simulink model "PWMepitettHidakhoz"  (R2013b)
settings: Solver=FixedStepDiscrete  SolverMode=SingleTasking  StartTime=0.0  StopTime=260000  FixedStep=0.1  RelTol=1e-3
undefined symbols (not defined in the file or in its folder): JA1, nexys2iroobo_lib
libraries: xbsIndex_r4 x41, simulink x2
settings Model: Creator=laca  LastModifiedBy=laca

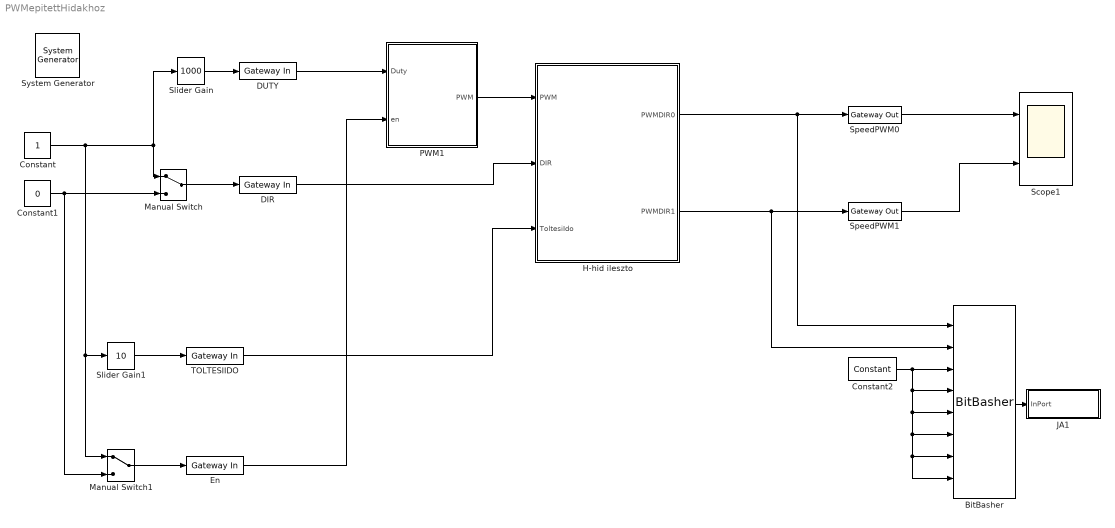
== system PWMepitettHidakhoz ==
  " System Generator" : xbsIndex_r4/ System Generator  Tag=genX  xilinxfamily=spartan3e  part=xc3s1200e  speed=-4  package=fg320  synthesis_tool=XST  clock_wrapper=Clock Enables  directory=./netlist  proj_type=Project Navigator  Synth_file=XST Defaults  Impl_file=ISE Defaults  testbench=off  simulink_period=1  sysclk_period=20  dcm_input_clock_period=10  incr_netlist=off  trim_vbits=Everywhere in SubSystem  dbl_ovrd=According to Block Masks  core_generation=According to Block Masks  run_coregen=off  deprecated_control=off  eval_field=0  block_type=sysgen
  BitBasher : xbsIndex_r4/BitBasher  bitexpr=|  display_expr=off  sr_1=1  arith_type1=Unsigned  bin_pt1=0  sr_2=2  arith_type2=Unsigned  bin_pt2=0  sr_3=3  arith_type3=Unsigned  bin_pt3=0  sr_4=4  arith_type4=Unsigned  bin_pt4=0  dbl_ovrd=off  block_type=bitbasher
      | <!DOCTYPE HTML PUBLIC "-//W3C//DTD HTML 4.0//EN" "http://www.w3.org/TR/REC-html40/strict.dtd">
      | <html><head><meta name="qrichtext" content="1" /><style type="text/css">
      | p, li { white-space: pre-wrap; }
      | </style></head><body style=" font-family:'MS Shell Dlg 2'; font-size:8.25pt; font-weight:400; font-style:normal;">
      | <p style=" margin-top:12px; margin-bottom:12px; margin-left:0px; margin-right:0px; -qt-block-indent:0; text-indent:0px;"><span style=" font-family:'MS Shell Dlg'; font-size:8pt;">a={b7,b6,b5,b4,b3,b2,b1,b0}</span></p></body></html>
  Constant : Constant
  Constant1 : Constant  Value=0
  Constant2 : xbsIndex_r4/Constant  const=0  gui_display_data_type=Boolean  arith_type=Boolean  n_bits=16  bin_pt=14  preci_type=Single  exp_width=8  frac_width=24  explicit_period=off  period=1  equ=P=C  opselect=C  inp2=PCIN>>17  opr=+  inp1=P  carry=CIN  dbl_ovrd=off  block_type=constant
  DIR : xbsIndex_r4/Gateway In  gui_display_data_type=Boolean  arith_type=Boolean  n_bits=16  bin_pt=0  preci_type=Single  exp_width=8  frac_width=24  quantization="Round  (unbiased: +/- Inf)"  overflow=Saturate  period=1  dbl_ovrd=off  timing_constraint=None  locs_specified=off  LOCs={}  UseAsADC=off  ADCChannel='1'  inherit_from_input=off  hdl_port=on  block_type=gatewayin
  DUTY : xbsIndex_r4/Gateway In  gui_display_data_type=Fixed-point  arith_type=Unsigned  n_bits=16  bin_pt=0  preci_type=Single  exp_width=8  frac_width=24  quantization="Round  (unbiased: +/- Inf)"  overflow=Saturate  period=1  dbl_ovrd=off  timing_constraint=None  locs_specified=off  LOCs={}  UseAsADC=off  ADCChannel='1'  inherit_from_input=off  hdl_port=on  block_type=gatewayin
  En : xbsIndex_r4/Gateway In  gui_display_data_type=Boolean  arith_type=Boolean  n_bits=16  bin_pt=14  preci_type=Single  exp_width=8  frac_width=24  quantization="Round  (unbiased: +/- Inf)"  overflow=Saturate  period=1  dbl_ovrd=off  timing_constraint=None  locs_specified=off  LOCs={}  UseAsADC=off  ADCChannel='1'  inherit_from_input=off  hdl_port=on  block_type=gatewayin
  H-hid ileszto : Subsystem
  JA1 : Subsystem  AncestorBlock=nexys2iroobo_lib/JA1  mask(Non-Memory-Mapped Output Port){show_out=off}
      mask prompts: show_out "Provide Output Double"
      mask help:
      | Port Name: "JA1"
      | Port Type: 8-bit Vector
      mask init:
      | [bg,fg] = xlcmap('IO',0);
      | iPos = get_param(gcb,'Position');
      | iWidth=iPos(3)-iPos(1);
      | iHeight=iPos(4)-iPos(2);
      | [logoX, logoY] = xlogo(iPos);
      | if (show_out)
      |     old = find_system(gcb, 'LookUnderMasks', 'all', 'Name', 'Terminator');
      |     if (length(old) > 0)
      |         replace_block(gcb, 'Name', 'Terminator', 'OutPort', 'noprompt');
      |         set_param([gcb '/Terminator'], 'Name', 'OutPort');
      |     end
      |     portdir = 'output';
      |     portstr = 'dbl';
      | else
      |     old = find_system(gcb, 'LookUnderMasks', 'all', 'name', 'OutPort');
      |     if (length(old) > 0)
      |         replace_block(gcb, 'Name', 'OutPort', 'Terminator', 'noprompt');
      |         set_param([gcb '/OutPort'], 'Name', 'Terminator');
      |     end
      |     portdir = 'input';
      |     portstr = '';
      | end
      settings: CopyFcn=set_param(gcb,'LinkStatus','inactive');
      mask Display:
      | patch([0 iWidth iWidth 0],[0 0 iHeight iHeight] , bg);
      | patch(logoX,logoY, fg);
      | plot([0 0 iWidth iWidth 0], [0 iHeight iHeight 0 0]);
      | port_label(portdir,1,portstr);
      | port_label('input',1,'JA1');
      | text(iWidth-10,5,'nmm');
  Manual Switch : ManualSwitch
  Manual Switch1 : ManualSwitch
  PWM1 : Subsystem
  Scope1 : Scope  NumInputPorts=2
      settings: TickLabels=on  ShowLegends=on  YMin=0~0  YMax=2000~1
  Slider Gain : simulink/Math Operations/Slider Gain  low=0  gain=1000  high=16535
  Slider Gain1 : simulink/Math Operations/Slider Gain  low=0  gain=10  high=1000
  SpeedPWM0 : xbsIndex_r4/Gateway Out  inherit_from_input=off  hdl_port=on  timing_constraint=None  locs_specified=off  LOCs={}  UseAsDAC=off  DACChannel='1'  block_type=gatewayout
      settings: xl_area=[0 0 0 0 1 0 0]
  SpeedPWM1 : xbsIndex_r4/Gateway Out  inherit_from_input=off  hdl_port=on  timing_constraint=None  locs_specified=off  LOCs={}  UseAsDAC=off  DACChannel='1'  block_type=gatewayout
      settings: xl_area=[0 0 0 0 1 0 0]
  TOLTESIIDO : xbsIndex_r4/Gateway In  gui_display_data_type=Fixed-point  arith_type=Unsigned  n_bits=16  bin_pt=0  preci_type=Single  exp_width=8  frac_width=24  quantization="Round  (unbiased: +/- Inf)"  overflow=Saturate  period=1  dbl_ovrd=off  timing_constraint=None  locs_specified=off  LOCs={}  UseAsADC=off  ADCChannel='1'  inherit_from_input=off  hdl_port=on  block_type=gatewayin
  wires:
  Manual Switch/1 -> DIR/1
  Slider Gain1/1 -> TOLTESIIDO/1
  TOLTESIIDO/1 -> H-hid ileszto/3(ToltesiIdo)
  Manual Switch1/1 -> En/1
  PWM1/1(PWM) -> H-hid ileszto/1(PWM)
  DIR/1 -> H-hid ileszto/2(DIR)
  H-hid ileszto/1(PWMDIR0) -> BitBasher/1, SpeedPWM0/1
  H-hid ileszto/2(PWMDIR1) -> BitBasher/2, SpeedPWM1/1
  En/1 -> PWM1/2(en)
  DUTY/1 -> PWM1/1(Duty)
  SpeedPWM0/1 -> Scope1/1
  SpeedPWM1/1 -> Scope1/2
  Slider Gain/1 -> DUTY/1
  Constant1/1 -> Manual Switch1/2, Manual Switch/2
  Constant/1 -> Slider Gain1/1, Manual Switch1/1, Slider Gain/1, Manual Switch/1
  BitBasher/1 -> JA1/1(InPort)
  Constant2/1 -> BitBasher/4, BitBasher/5, BitBasher/6, BitBasher/7, BitBasher/8, BitBasher/3

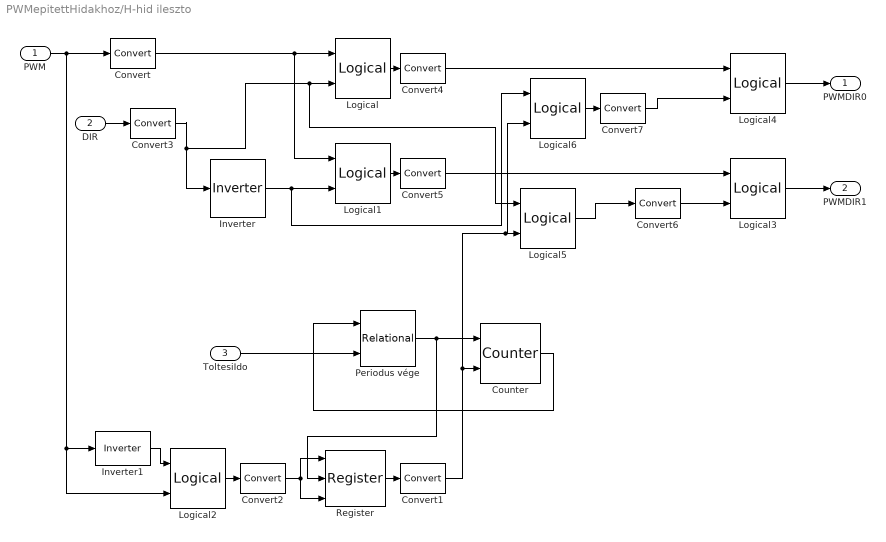
== system PWMepitettHidakhoz/H-hid ileszto ==
  PWM : Inport
  DIR : Inport  Port=2
  ToltesiIdo : Inport  Port=3
  Convert{,1..7} (8 alike) : xbsIndex_r4/Convert  gui_display_data_type=Boolean  arith_type=Boolean  n_bits=16  bin_pt=14  float_type=Single  exp_bits=8  fraction_bits=24  quantization=Truncate  overflow=Wrap  en=off  latency=0  dbl_ovrd=off  pipeline=off  block_type=convert
  Counter : xbsIndex_r4/Counter  cnt_type=Free Running  cnt_to=Inf  operation=Up  start_count=0  cnt_by_val=1  arith_type=Unsigned  n_bits=16  bin_pt=0  load_pin=off  rst=on  en=on  explicit_period=off  period=2*10^-2  dbl_ovrd=off  use_behavioral_HDL=off  implementation=Fabric  block_type=counter
  Inverter : xbsIndex_r4/Inverter  en=off  latency=0  dbl_ovrd=off  block_type=inv
  Inverter1 : xbsIndex_r4/Inverter  en=off  latency=1  dbl_ovrd=off  block_type=inv
  Logical{,1..2,5..6} (5 alike) : xbsIndex_r4/Logical  logical_function=AND  inputs=2  en=off  latency=0  precision=User Defined  arith_type=Unsigned  n_bits=1  bin_pt=0  align_bp=on  dbl_ovrd=off  block_type=logical
  Logical3 : xbsIndex_r4/Logical  logical_function=OR  inputs=2  en=off  latency=0  precision=User Defined  arith_type=Unsigned  n_bits=1  bin_pt=0  align_bp=on  dbl_ovrd=off  block_type=logical
  Logical4 : xbsIndex_r4/Logical  logical_function=OR  inputs=2  en=off  latency=0  precision=User Defined  arith_type=Unsigned  n_bits=1  bin_pt=0  align_bp=on  dbl_ovrd=off  block_type=logical
  Periodus vége : xbsIndex_r4/Relational  mode=a=b  en=off  latency=0  dbl_ovrd=off  block_type=relational
  Register : xbsIndex_r4/Register  init=0  rst=on  en=on  dbl_ovrd=off  block_type=register
  PWMDIR0 : Outport
  PWMDIR1 : Outport  Port=2
  wires:
  DIR/1 -> Convert3/1
  Inverter/1 -> Logical6/1, Logical1/2
  Convert/1 -> Logical1/1, Logical/1
  Counter/1 -> Periodus vége/1
  Periodus vége/1 -> Register/2, Counter/1
  ToltesiIdo/1 -> Periodus vége/2
  PWM/1 -> Convert/1, Logical2/2, Inverter1/1
  Inverter1/1 -> Logical2/1
  Logical2/1 -> Convert2/1
  Logical3/1 -> PWMDIR1/1
  Logical1/1 -> Convert5/1
  Logical4/1 -> PWMDIR0/1
  Logical/1 -> Convert4/1
  Register/1 -> Convert1/1
  Convert1/1 -> Logical6/2, Logical5/2, Counter/2
  Convert2/1 -> Register/3, Register/1
  Convert3/1 -> Inverter/1, Logical5/1, Logical/2
  Convert4/1 -> Logical4/1
  Convert5/1 -> Logical3/1
  Logical5/1 -> Convert6/1
  Logical6/1 -> Convert7/1
  Convert6/1 -> Logical3/2
  Convert7/1 -> Logical4/2

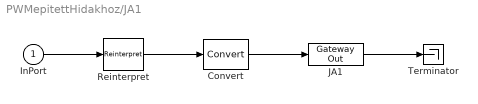
== system PWMepitettHidakhoz/JA1 ==
  InPort : Inport
  Convert : xbsIndex_r4/Convert  gui_display_data_type=Fixed-point  arith_type=Unsigned  n_bits=8  bin_pt=0  float_type=Single  exp_bits=8  fraction_bits=24  quantization=Truncate  overflow=Wrap  en=off  latency=0  dbl_ovrd=off  pipeline=off  block_type=convert
  JA1 : xbsIndex_r4/Gateway Out  inherit_from_input=off  hdl_port=on  timing_constraint=None  locs_specified=on  LOCs={'M16','M14','L16','K13','M15','L17','K12','L15'}  UseAsDAC=off  DACChannel='1'  block_type=gatewayout
      settings: sginterface={'Xilinx'=>{'jtaghwcosim'=>{'non_memory_mapped_port'=>'JA1'}}}
  Reinterpret : xbsIndex_r4/Reinterpret  force_arith_type=off  arith_type=Unsigned  force_bin_pt=off  bin_pt=0  block_type=reinterpret
  Terminator : Terminator
  wires:
  JA1/1 -> Terminator/1
  Convert/1 -> JA1/1
  Reinterpret/1 -> Convert/1
  InPort/1 -> Reinterpret/1

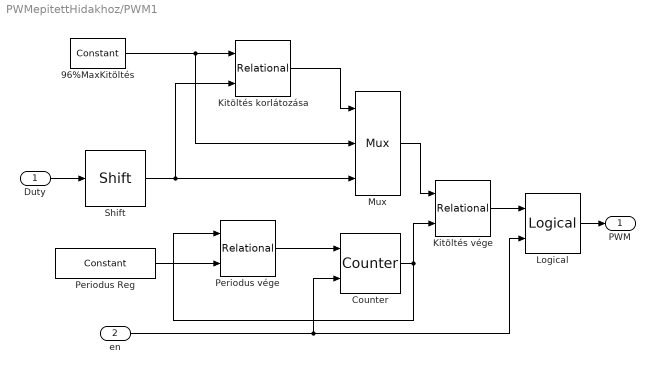
== system PWMepitettHidakhoz/PWM1 ==
  Duty : Inport
  en : Inport  Port=2
  96%MaxKitöltés : xbsIndex_r4/Constant  const=15800  gui_display_data_type=Fixed-point  arith_type=Unsigned  n_bits=16  bin_pt=0  preci_type=Single  exp_width=8  frac_width=24  explicit_period=off  period=1  equ=P=C  opselect=C  inp2=PCIN>>17  opr=+  inp1=P  carry=CIN  dbl_ovrd=off  block_type=constant
  Counter : xbsIndex_r4/Counter  cnt_type=Free Running  cnt_to=Inf  operation=Up  start_count=0  cnt_by_val=1  arith_type=Unsigned  n_bits=16  bin_pt=0  load_pin=off  rst=on  en=on  explicit_period=off  period=2*10^-2  dbl_ovrd=off  use_behavioral_HDL=off  implementation=Fabric  block_type=counter
  Kitöltés vége : xbsIndex_r4/Relational  mode=a>b  en=off  latency=0  dbl_ovrd=off  block_type=relational
  Kitöltés korlátozása : xbsIndex_r4/Relational  mode=a>b  en=off  latency=0  dbl_ovrd=off  block_type=relational
  Logical : xbsIndex_r4/Logical  logical_function=AND  inputs=2  en=off  latency=0  precision=User Defined  arith_type=Unsigned  n_bits=1  bin_pt=0  align_bp=on  dbl_ovrd=off  block_type=logical
  Mux : xbsIndex_r4/Mux  inputs=2  en=off  latency=0  precision=User Defined  arith_type=Unsigned  n_bits=16  bin_pt=0  quantization=Truncate  overflow=Wrap  dbl_ovrd=off  block_type=mux
  Periodus vége : xbsIndex_r4/Relational  mode=a=b  en=off  latency=0  dbl_ovrd=off  block_type=relational
  Periodus Reg : xbsIndex_r4/Constant  const=16383  gui_display_data_type=Fixed-point  arith_type=Unsigned  n_bits=17  bin_pt=0  preci_type=Single  exp_width=8  frac_width=24  explicit_period=on  period=1  equ=P=C  opselect=C  inp2=PCIN>>17  opr=+  inp1=P  carry=CIN  dbl_ovrd=off  block_type=constant
  Shift : xbsIndex_r4/Shift  shift_dir=Right  shift_bits=2  en=off  latency=0  precision=User Defined  arith_type="Signed  (2's comp)"  n_bits=16  bin_pt=0  quantization=Truncate  overflow=Saturate  dbl_ovrd=off  block_type=shift
  PWM : Outport
  wires:
  Counter/1 -> Periodus vége/1, Kitöltés vége/2
  Periodus vége/1 -> Counter/1
  en/1 -> Logical/2, Counter/2
  Kitöltés vége/1 -> Logical/1
  Logical/1 -> PWM/1
  Duty/1 -> Shift/1
  Periodus Reg/1 -> Periodus vége/2
  96%MaxKitöltés/1 -> Mux/2, Kitöltés korlátozása/1
  Mux/1 -> Kitöltés vége/1
  Kitöltés korlátozása/1 -> Mux/1
  Shift/1 -> Mux/3, Kitöltés korlátozása/2
